simulink model "Vx_K23"  (R2018b)
settings: Solver=ode45  StartTime=0.0  StopTime=200  RelTol=1e-3  EnableMultiTasking=on
values from neighbouring files (symbols this model uses):
  K = lqr(Ap,Bp,Q,R)    [ControllerDesign.m]    (also in MatrixSetup_Fixed.m; TunedControlSystem.m)
undefined symbols (not defined in the file or in its folder): Advantech, PCI
libraries: sldrtlib x3, simulink x1
settings Model: ExtModeTrigMode=oneshot  ExtModeArmWhenConnect=off  Creator=qqgarcia  LastModifiedBy=nedunash
settings DataIOCC: SaveFormat=Array  SignalLoggingSaveFormat=ModelDataLogs  SaveOutput=off  SaveTime=off
settings OptimizationCC: BlockReduction=off  BooleanDataType=off  ExpressionDepthLimit=2147483647  InitFltsAndDblsToZero=on  LifeSpan=inf
settings DebuggingCC: SaveWithParameterizedLinksMsg=none  UnderspecifiedInitializationDetection=Classic  MergeDetectMultiDrivingBlocksExec=none  SignalResolutionControl=TryResolveAllWithWarning  MultiTaskDSMMsg=warning  MultiTaskCondExecSysMsg=none  FcnCallInpInsideContextMsg=warning  StateNameClashWarn=warning  SFUnexpectedBacktrackingDiag=warning  SFNoUnconditionalDefaultTransitionDiag=warning  SFExecutionAtInitializationDiag=none
settings HardwareCC: ProdBitPerPointer=32  ProdBitPerSizeT=32  ProdBitPerPtrDiffT=32  ProdLargestAtomicFloat=None  ProdIntDivRoundTo=Undefined  ProdEndianess=Unspecified  ProdWordSize=32  ProdHWDeviceType=32-bit Generic  TargetUnknown=on
settings ModelReferenceCC: PropagateSignalLabelsOutOfModel=off
settings SFSimCC: SimUseLocalCustomCode=off
settings RTWCC: RTWUseLocalCustomCode=off
settings CodeAppCC: StateflowObjectComments=on
settings GRTTargetCC: TargetFcnLib=ansi_tfl_tmw.mat  TargetLangStandard=C89/C90 (ANSI)  GeneratePreprocessorConditionals=Disable all  CombineOutputUpdateFcns=off  GRTInterface=on
settings ConfigComp: CovMetricSettings=dw  CovHtmlReporting=on  CovSaveCumulativeToWorkspaceVar=on  CovSaveSingleToWorkspaceVar=on  CovExternalEMLEnable=off  CovSFcnEnable=off

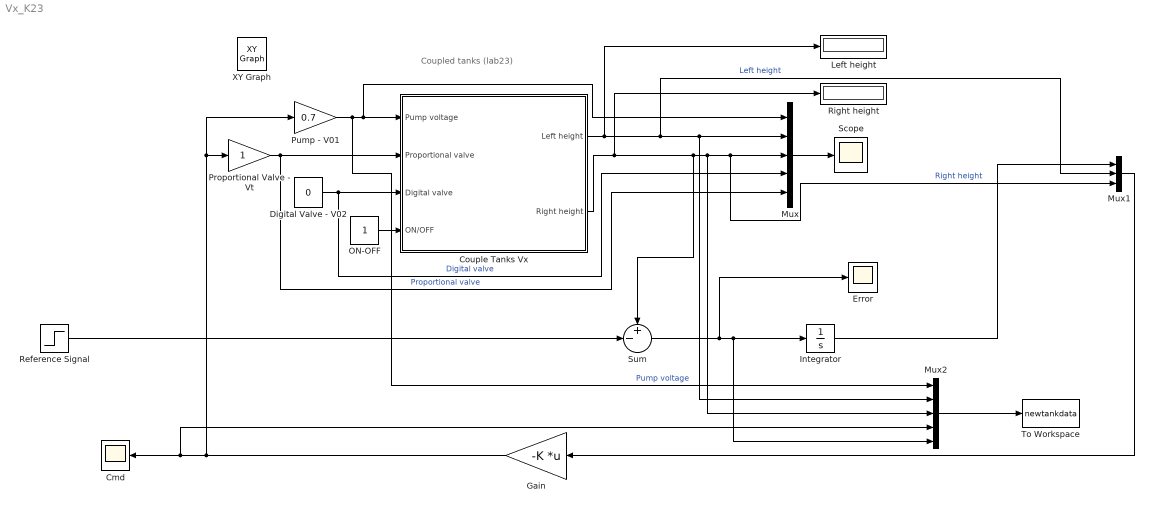
== system Vx_K23 ==
  note: Coupled tanks (lab23)
  Cmd : Scope
  Couple Tanks Vx : Subsystem  mask(Tanks){Ts=0.1}
      mask prompts: Ts "Sampling Time {Ts = 0.12 s;  0.05 - 0.5 s}"
      mask help: Vodarna Vx K23
      mask Help: Ovlada model vodarny. Periodu vzorkovani Ts volte v rozsahu 0.05 s < Ts < 0.5 s (doporucena Ts = 0.12 s).  Merena data jsou filtrovana dolnofrekvencnim filtrem (Butterworth druhy rad s pasmovou frekvenci w = 2 rad/s)  a ukladana po radcich do matice ty v pracovnim prostoru Matlabu. Prvni sloupec matice ty predstavuje cas a dalsi pak jednotlive promenne v poradi vstupu do bloku multiplexoru osciloskopu.     (JF2000-2007)
      mask Display: image(imread('Vxpic.tif'))
  Digital Valve - V02 : Constant  Value=0
  Error : Scope
  Gain : Gain  Gain=-K  Multiplication=Matrix(K*u)
  Integrator : Integrator
  Left height : Display
      settings: SampleTime=2
  Mux : Mux  Inputs=5
  Mux1 : Mux  Inputs=3
  Mux2 : Mux  Inputs=5
  ON-OFF : Constant
  Proportional Valve - Vt : Gain
  Pump - V01 : Gain  Gain=0.7
  Reference Signal : Step  Time=0  After=0.18  SampleTime=60
  Right height : Display
      settings: SampleTime=2
  Scope : Scope
  Sum : Sum  Inputs=+-|
  To Workspace : ToWorkspace  VariableName=newtankdata  SaveFormat=Timeseries  SampleTime=-1
  XY Graph : simulink/Sinks/XY Graph  IOType=viewer  xmin=-1  xmax=1  ymin=-1  ymax=1  st=-1
  wires:
  Pump - V01/1 -> Mux2/1, Couple Tanks Vx/1(Pump voltage), Mux/1  "Pump voltage"
  Proportional Valve - Vt/1 -> Mux/5, Couple Tanks Vx/2(Proportional valve)  "Proportional valve"
  ON-OFF/1 -> Couple Tanks Vx/4(ON/OFF)
  Couple Tanks Vx/1(Left height) -> Mux1/2, Mux2/2, Mux/2, Left height/1  "Left height"
  Digital Valve - V02/1 -> Mux/4, Couple Tanks Vx/3(Digital valve)  "Digital valve"
  Couple Tanks Vx/2(Right height) -> Sum/1, Mux2/3, Mux1/3, Mux/3, Right height/1  "Right height"
  Mux/1 -> Scope/1
  Sum/1 -> Error/1, Mux2/5, Integrator/1
  Reference Signal/1 -> Sum/2
  Mux1/1 -> Gain/1
  Integrator/1 -> Mux1/1
  Mux2/1 -> To Workspace/1
  Gain/1 -> Mux2/4, Cmd/1, Proportional Valve - Vt/1, Pump - V01/1

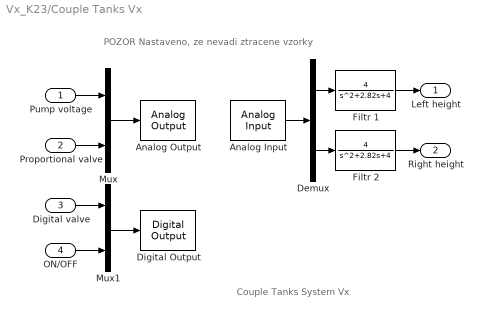
== system Vx_K23/Couple Tanks Vx ==
  note: Couple Tanks System Vx
  note: POZOR Nastaveno, ze nevadi ztracene vzorky
  Pump voltage : Inport
  Proportional valve : Inport  Port=2
  Digital valve : Inport  Port=3
  ON/OFF : Inport  Port=4
  Analog Input : sldrtlib/Analog Input  SampleTime=Ts  MaxMissedTicks=1000  ShowMissedTicks=off  YieldWhenWaiting=on  DrvName=Advantech/PCI-1711  DrvAddress=4294967295  DrvOptions=zeros(1,0)  Channels=1:2  RangeMode=2  VoltRange=1  DataType=1
      settings: AttributesFormatString=Advantech\nPCI-1711 [auto]  SourceProductName=Simulink Desktop Real-Time
  Analog Output : sldrtlib/Analog Output  SampleTime=Ts  MaxMissedTicks=1000  ShowMissedTicks=off  YieldWhenWaiting=on  DrvName=Advantech/PCI-1711  DrvAddress=4294967295  DrvOptions=zeros(1,0)  Channels=1:2  RangeMode=3  VoltRange=2  InitialValue=[0 0]  FinalValue=[0 0]
      settings: AttributesFormatString=Advantech\nPCI-1711 [auto]  SourceProductName=Simulink Desktop Real-Time
  Demux : Demux  Outputs=2
  Digital Output : sldrtlib/Digital Output  SampleTime=Ts  MaxMissedTicks=1000  ShowMissedTicks=off  YieldWhenWaiting=on  DrvName=Advantech/PCI-1711  DrvAddress=4294967295  DrvOptions=zeros(1,0)  Channels=[2 1]  BitMode=1  InitialValue=[0 1]  FinalValue=[0 0]
      settings: AttributesFormatString=Advantech\nPCI-1711 [auto]  SourceProductName=Simulink Desktop Real-Time  SourceProductBaseCode=WT
  Filtr 1 : TransferFcn  Numerator=[4]  Denominator=[1 2.82 4]
  Filtr 2 : TransferFcn  Numerator=[4]  Denominator=[1 2.82 4]
  Mux : Mux  Inputs=2
  Mux1 : Mux  Inputs=2
  Left height : Outport
  Right height : Outport  Port=2
  wires:
  Analog Input/1 -> Demux/1
  Mux/1 -> Analog Output/1
  Digital valve/1 -> Mux1/1
  ON/OFF/1 -> Mux1/2
  Mux1/1 -> Digital Output/1
  Pump voltage/1 -> Mux/1
  Proportional valve/1 -> Mux/2
  Demux/1 -> Filtr 1/1
  Demux/2 -> Filtr 2/1
  Filtr 1/1 -> Left height/1
  Filtr 2/1 -> Right height/1
